simulink model "lab7"  (R2021b)
settings: Solver=ode45  StartTime=0.0  StopTime=250  RelTol=1e-3  EnableMultiTasking=on
values from neighbouring files (symbols this model uses):
  ddMax = 3    [sysdata.m]
  deltaMax = 30    [sysdata.m]
  fConst = 0    [sysdata.m]
  K = 0.08    [lab2_otay.m]    (also in sysdata.m)
  Kaw = 8.1280    (= 8.128)    [lab6go.m]    (also in lab7go.m)
  Kc = 0.825    [sysdata.m]
  phiZad = 90    [sysdata.m]
  T = aT(i)    [lab7go.m]
  TI = 200    [sysdata.m]
  Toc = 5    [lab2_otay.m]    (also in sysdata.m)
  TR = 1    [lab2_otay.m]    (also in sysdata.m)
  Ts = 18.0    (= 18)    [lab2_otay.m]    (also in sysdata.m)
undefined symbols (not defined in the file or in its folder): dD, nD
settings Model: Creator=user  LastModifiedBy=Lapte
settings SolverCC: AlgebraicLoopSolver=TrustRegion
settings DataIOCC: LimitDataPoints=on  SaveFormat=Array  ReturnWorkspaceOutputs=off
settings OptimizationCC: LifeSpan=inf
settings DebuggingCC: SFUnexpectedBacktrackingDiag=warning  SFNoUnconditionalDefaultTransitionDiag=warning  SFExecutionAtInitializationDiag=none  SFMachineParentedDataDiag=warning  ArithmeticOperatorsInVariantConditions=warning
settings HardwareCC: ProdBitPerPointer=32  ProdBitPerSizeT=32  ProdBitPerPtrDiffT=32  ProdLargestAtomicFloat=None  ProdIntDivRoundTo=Undefined  ProdEndianess=Unspecified  ProdWordSize=32  ProdHWDeviceType=32-bit Generic
settings ModelReferenceCC: PropagateSignalLabelsOutOfModel=off
settings SFSimCC: SimUseLocalCustomCode=off  CustomCodeUndefinedFunction=UseInterfaceOnly
settings RTWCC: RTWUseLocalCustomCode=off
settings CodeAppCC: StateflowObjectComments=on
settings GRTTargetCC: TargetLangStandard=C89/C90 (ANSI)
settings ConfigComp: CovMetricSettings=dw  CovSaveCumulativeToWorkspaceVar=on  CovSaveSingleToWorkspaceVar=on  CovExternalEMLEnable=off  CovSFcnEnable=off

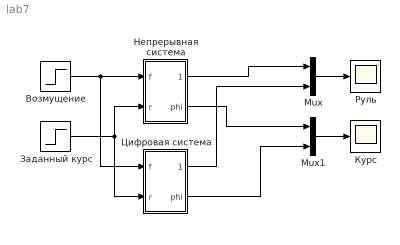
== system lab7 ==
  Mux : Mux  Inputs=2
  Mux1 : Mux  Inputs=2
  Возмущение : Step  Time=0  After=fConst  SampleTime=0
  Заданный курс : Step  Time=0  After=phiZad  SampleTime=0
  Курс : Scope
  Непрерывная система : Subsystem
  Руль : Scope
  Цифровая система : Subsystem
  wires:
  Возмущение/1 -> Цифровая система/1(f), Непрерывная система/1(f)
  Заданный курс/1 -> Непрерывная система/2(r), Цифровая система/2(r)
  Непрерывная система/1(delta) -> Mux/1
  Непрерывная система/2(phi) -> Mux1/1
  Mux/1 -> Руль/1
  Mux1/1 -> Курс/1
  Цифровая система/1(delta) -> Mux/2
  Цифровая система/2(phi) -> Mux1/2

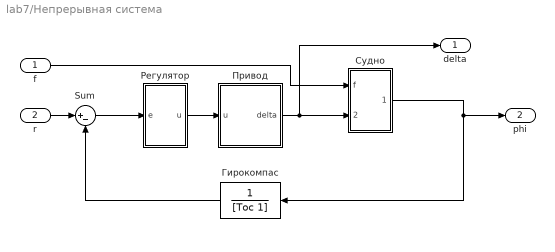
== system lab7/Непрерывная система ==
  f : Inport
  r : Inport  Port=2
  Sum : Sum  Inputs=|+-
  Гирокомпас : TransferFcn  Denominator=[Toc 1]
  Привод : Subsystem
  Регулятор : Subsystem
  Судно : Subsystem
  delta : Outport
  phi : Outport  Port=2
  wires:
  f/1 -> Судно/1(f)
  r/1 -> Sum/1
  Привод/1(delta) -> Судно/2(delta), delta/1
  Sum/1 -> Регулятор/1(e)
  Гирокомпас/1 -> Sum/2
  Судно/1(phi) -> Гирокомпас/1, phi/1
  Регулятор/1(u) -> Привод/1(u)

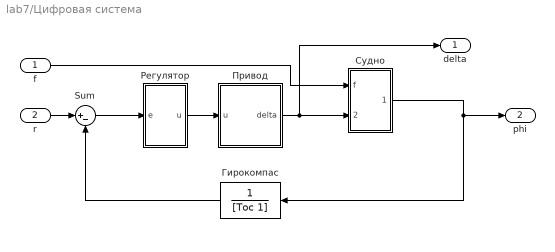
== system lab7/Цифровая система ==
  f : Inport
  r : Inport  Port=2
  Sum : Sum  Inputs=|+-
  Гирокомпас : TransferFcn  Denominator=[Toc 1]
  Привод : Subsystem
  Регулятор : Subsystem
  Судно : Subsystem
  delta : Outport
  phi : Outport  Port=2
  wires:
  Регулятор/1(u) -> Привод/1(u)
  Судно/1(phi) -> phi/1, Гирокомпас/1
  Гирокомпас/1 -> Sum/2
  Sum/1 -> Регулятор/1(e)
  Привод/1(delta) -> delta/1, Судно/2(delta)
  r/1 -> Sum/1
  f/1 -> Судно/1(f)

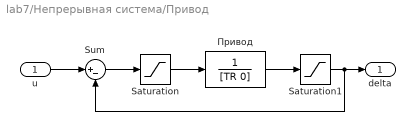
== system lab7/Непрерывная система/Привод ==
  u : Inport
  Saturation : Saturate  UpperLimit=TR*ddMax  LowerLimit=-TR*ddMax
  Saturation1 : Saturate  UpperLimit=deltaMax  LowerLimit=-deltaMax
  Sum : Sum  Inputs=|+-
  Привод : TransferFcn  Denominator=[TR 0]
  delta : Outport
  wires:
  Sum/1 -> Saturation/1
  u/1 -> Sum/1
  Saturation/1 -> Привод/1
  Привод/1 -> Saturation1/1
  Saturation1/1 -> delta/1, Sum/2

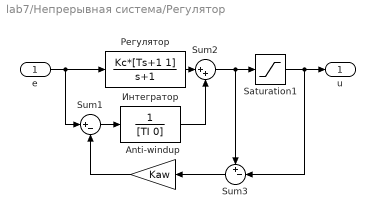
== system lab7/Непрерывная система/Регулятор ==
  e : Inport
  Anti-windup : Gain  Gain=Kaw
  Saturation1 : Saturate  UpperLimit=deltaMax  LowerLimit=-deltaMax
  Sum1 : Sum  Inputs=|+-
  Sum2 : Sum  Inputs=|++
  Sum3 : Sum  Inputs=+-|
  Интегратор : TransferFcn  Denominator=[TI 0]
  Регулятор : TransferFcn  Numerator=Kc*[Ts+1 1]  Denominator=[1 1]
  u : Outport
  wires:
  Регулятор/1 -> Sum2/1
  e/1 -> Sum1/1, Регулятор/1
  Интегратор/1 -> Sum2/2
  Sum1/1 -> Интегратор/1
  Saturation1/1 -> u/1, Sum3/2
  Sum2/1 -> Sum3/1, Saturation1/1
  Sum3/1 -> Anti-windup/1
  Anti-windup/1 -> Sum1/2

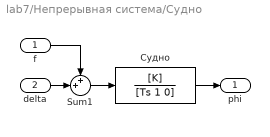
== system lab7/Непрерывная система/Судно ==
  f : Inport
  delta : Inport  Port=2
  Sum1 : Sum  Inputs=++|
  Судно : TransferFcn  Numerator=[K]  Denominator=[Ts 1 0]
  phi : Outport
  wires:
  Судно/1 -> phi/1
  f/1 -> Sum1/1
  Sum1/1 -> Судно/1
  delta/1 -> Sum1/2

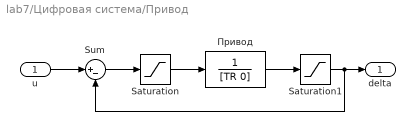
== system lab7/Цифровая система/Привод ==
  u : Inport
  Saturation : Saturate  UpperLimit=TR*ddMax  LowerLimit=-TR*ddMax
  Saturation1 : Saturate  UpperLimit=deltaMax  LowerLimit=-deltaMax
  Sum : Sum  Inputs=|+-
  Привод : TransferFcn  Denominator=[TR 0]
  delta : Outport
  wires:
  Saturation1/1 -> Sum/2, delta/1
  Привод/1 -> Saturation1/1
  Saturation/1 -> Привод/1
  u/1 -> Sum/1
  Sum/1 -> Saturation/1

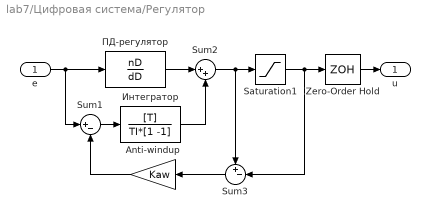
== system lab7/Цифровая система/Регулятор ==
  e : Inport
  Anti-windup : Gain  Gain=Kaw
  Saturation1 : Saturate  UpperLimit=deltaMax  LowerLimit=-deltaMax
  Sum1 : Sum  Inputs=|+-
  Sum2 : Sum  Inputs=|++
  Sum3 : Sum  Inputs=+-|
  Zero-Order Hold : ZeroOrderHold  SampleTime=T
  Интегратор : DiscreteTransferFcn  Numerator=[T]  Denominator=TI*[1 -1]  SampleTime=T
  ПД-регулятор : DiscreteTransferFcn  Numerator=nD  Denominator=dD  SampleTime=T
  u : Outport
  wires:
  Anti-windup/1 -> Sum1/2
  Sum3/1 -> Anti-windup/1
  Sum2/1 -> Saturation1/1, Sum3/1
  Saturation1/1 -> Zero-Order Hold/1, Sum3/2
  Sum1/1 -> Интегратор/1
  Интегратор/1 -> Sum2/2
  e/1 -> ПД-регулятор/1, Sum1/1
  ПД-регулятор/1 -> Sum2/1
  Zero-Order Hold/1 -> u/1

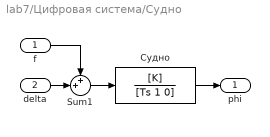
== system lab7/Цифровая система/Судно ==
  f : Inport
  delta : Inport  Port=2
  Sum1 : Sum  Inputs=++|
  Судно : TransferFcn  Numerator=[K]  Denominator=[Ts 1 0]
  phi : Outport
  wires:
  delta/1 -> Sum1/2
  Sum1/1 -> Судно/1
  f/1 -> Sum1/1
  Судно/1 -> phi/1
